simulink model "lab5"  (R2019b)
settings: Solver=VariableStepAuto  StartTime=0.0  StopTime=50.0  RelTol=1e-3
settings Model: Creator=Michał  LastModifiedBy=Michał

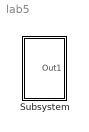
== system lab5 ==
  Subsystem : Subsystem  mask{r=2, Rd=0.001, th=90, vr=0, vth=0, g=9.81, m1=1, M=1, m2=1.4}
      mask prompts: Rd "R"; vth "vrh"

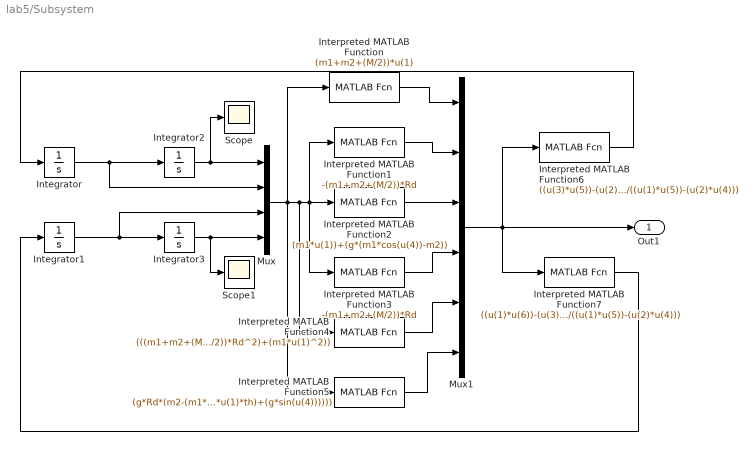
== system lab5/Subsystem ==
  Integrator : Integrator  InitialCondition=vr
  Integrator1 : Integrator  InitialCondition=vth
  Integrator2 : Integrator  InitialCondition=r
  Integrator3 : Integrator  InitialCondition=th*(pi/180)
  Interpreted MATLAB Function : MATLABFcn  MATLABFcn=(m1+m2+(M/2))*u(1)  OutputDimensions=1
  Interpreted MATLAB Function1 : MATLABFcn  MATLABFcn=-(m1+m2+(M/2))*Rd  OutputDimensions=1
  Interpreted MATLAB Function2 : MATLABFcn  MATLABFcn=(m1*u(1))+(g*(m1*cos(u(4))-m2))  OutputDimensions=1
  Interpreted MATLAB Function3 : MATLABFcn  MATLABFcn=-(m1+m2+(M/2))*Rd  OutputDimensions=1
  Interpreted MATLAB Function4 : MATLABFcn  MATLABFcn=(((m1+m2+(M/2))*Rd^2)+(m1*u(1)^2))  OutputDimensions=1
  Interpreted MATLAB Function5 : MATLABFcn  MATLABFcn=(g*Rd*(m2-(m1*cos(u(4)))) - (m1*r*((2*u(1)*th)+(g*sin(u(4))))))  OutputDimensions=1
  Interpreted MATLAB Function6 : MATLABFcn  MATLABFcn=((u(3)*u(5))-(u(2)*u(6)))/((u(1)*u(5))-(u(2)*u(4)))  OutputDimensions=1
  Interpreted MATLAB Function7 : MATLABFcn  MATLABFcn=((u(1)*u(6))-(u(3)*u(4)))/((u(1)*u(5))-(u(2)*u(4)))  OutputDimensions=1
  Mux : Mux
  Mux1 : Mux  Inputs=6
  Scope : Scope
  Scope1 : Scope
  Out1 : Outport
  wires:
  Interpreted MATLAB Function6/1 -> Integrator/1
  Integrator3/1 -> Scope1/1, Mux/4
  Integrator2/1 -> Scope/1, Mux/1
  Mux/1 -> Interpreted MATLAB Function5/1, Interpreted MATLAB Function/1, Interpreted MATLAB Function4/1, Interpreted MATLAB Function3/1, Interpreted MATLAB Function1/1, Interpreted MATLAB Function2/1
  Integrator1/1 -> Integrator3/1, Mux/3
  Interpreted MATLAB Function3/1 -> Mux1/4
  Integrator/1 -> Mux/2, Integrator2/1
  Mux1/1 -> Interpreted MATLAB Function6/1, Out1/1, Interpreted MATLAB Function7/1
  Interpreted MATLAB Function1/1 -> Mux1/2
  Interpreted MATLAB Function5/1 -> Mux1/6
  Interpreted MATLAB Function/1 -> Mux1/1
  Interpreted MATLAB Function7/1 -> Integrator1/1
  Interpreted MATLAB Function4/1 -> Mux1/5
  Interpreted MATLAB Function2/1 -> Mux1/3
